simulink model "Calc"  (R2021a)
settings: Solver=VariableStepAuto  StartTime=0.0  StopTime=10.0  RelTol=1e-3
libraries: simulink x3
settings Model: Creator=Ms store  LastModifiedBy=Ms store

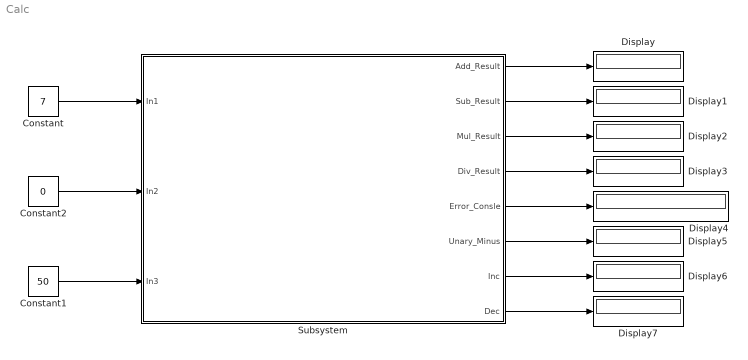
== system Calc ==
  Constant : Constant  Value=7
  Constant1 : Constant  Value=50
  Constant2 : Constant  Value=0
  Display{,1..7} (8 alike) : Display
  Subsystem : Subsystem
  wires:
  Constant/1 -> Subsystem/1(In1)
  Constant2/1 -> Subsystem/2(In2)
  Constant1/1 -> Subsystem/3(In3)
  Subsystem/1(Add_Result) -> Display/1
  Subsystem/2(Sub_Result) -> Display1/1
  Subsystem/3(Mul_Result) -> Display2/1
  Subsystem/4(Div_Result) -> Display3/1
  Subsystem/5(Error_Consle) -> Display4/1
  Subsystem/6(Unary_Minus) -> Display5/1
  Subsystem/7(Inc) -> Display6/1
  Subsystem/8(Dec) -> Display7/1

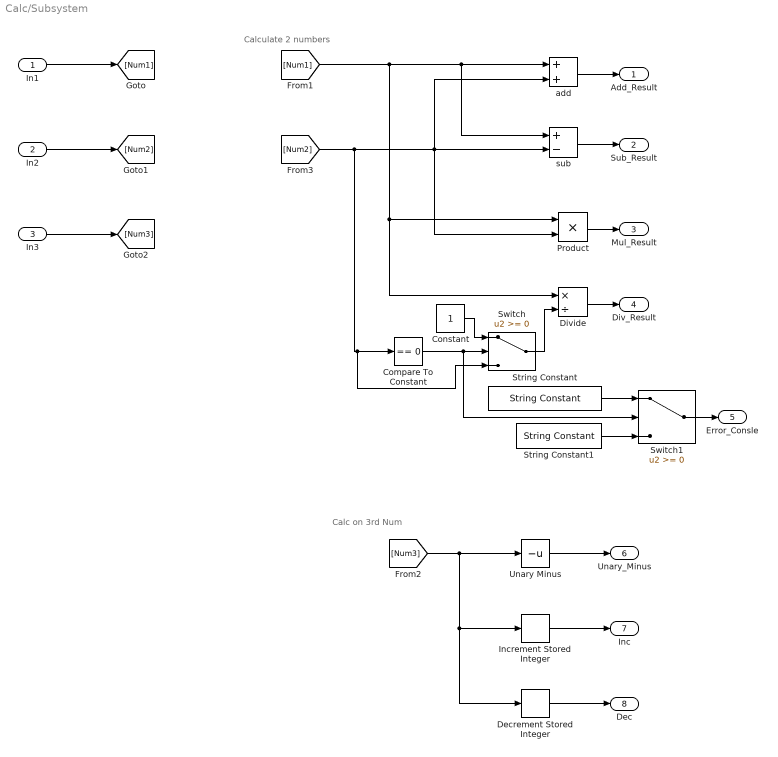
== system Calc/Subsystem ==
  note: Calc on 3rd Num
  note: Calculate 2 numbers
  In1 : Inport
  In2 : Inport  Port=2
  In3 : Inport  Port=3
  Compare To Constant : simulink/Logic and Bit Operations/Compare To Constant  relop===  const=0  OutDataTypeStr=boolean
  Constant : Constant
  Decrement Stored Integer : simulink/Additional Math & Discrete/Additional Math: Increment - Decrement/Decrement Stored Integer
      settings: SourceProductBaseCode=SL
  Divide : Product  Inputs=*/
  Increment Stored Integer : simulink/Additional Math & Discrete/Additional Math: Increment - Decrement/Increment Stored Integer
  Product : Product
  String Constant : StringConstant  String="\"Error, Division by Zero\""
  String Constant1 : StringConstant  String="\"Division Passed\""
  Switch : Switch
  Switch1 : Switch
  Unary Minus : UnaryMinus
  add : Sum
  sub : Sum  Inputs=+-
  Add_Result : Outport
  Sub_Result : Outport  Port=2
  Mul_Result : Outport  Port=3
  Div_Result : Outport  Port=4
  Error_Consle : Outport  Port=5
  Unary_Minus : Outport  Port=6
  Inc : Outport  Port=7
  Dec : Outport  Port=8
  wires:
  In1/1 -> [Num1]
  In2/1 -> [Num2]
  In3/1 -> [Num3]
  [Num1] -> Divide/1, Product/1, sub/1, add/1
  add/1 -> Add_Result/1
  [Num2] -> Switch/3, Compare To Constant/1, sub/2, add/2, Product/2
  sub/1 -> Sub_Result/1
  Product/1 -> Mul_Result/1
  Compare To Constant/1 -> Switch1/2, Switch/2
  Switch/1 -> Divide/2
  Divide/1 -> Div_Result/1
  Constant/1 -> Switch/1
  String Constant/1 -> Switch1/1
  String Constant1/1 -> Switch1/3
  Switch1/1 -> Error_Consle/1
  [Num3] -> Decrement Stored Integer/1, Increment Stored Integer/1, Unary Minus/1
  Unary Minus/1 -> Unary_Minus/1
  Increment Stored Integer/1 -> Inc/1
  Decrement Stored Integer/1 -> Dec/1
